simulink model "sampleModel106"  (R2022a)
settings: Solver=VariableStepAuto  StartTime=0.0  StopTime=10.0  RelTol=1e-3
undefined symbols (not defined in the file): DiscIntNeverNeededParam, magnitude, Newton, Raphson
libraries: simulink x379, slpidlib x89
(part 1 of 16)
settings Model: Creator=user  LastModifiedBy=CMelt
settings SolverCC: ZeroCrossControl=DisableAll

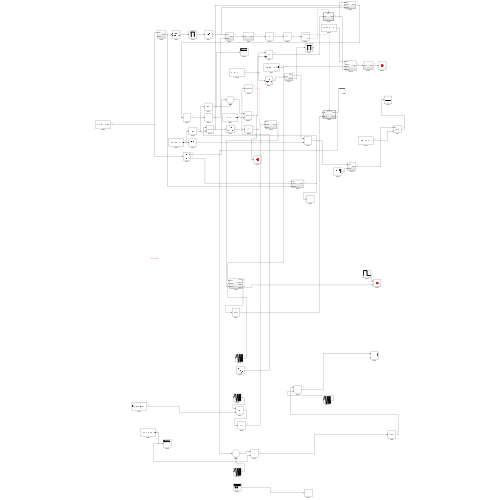
[thumbnail: Simulink's stored preview of the top-level diagram]
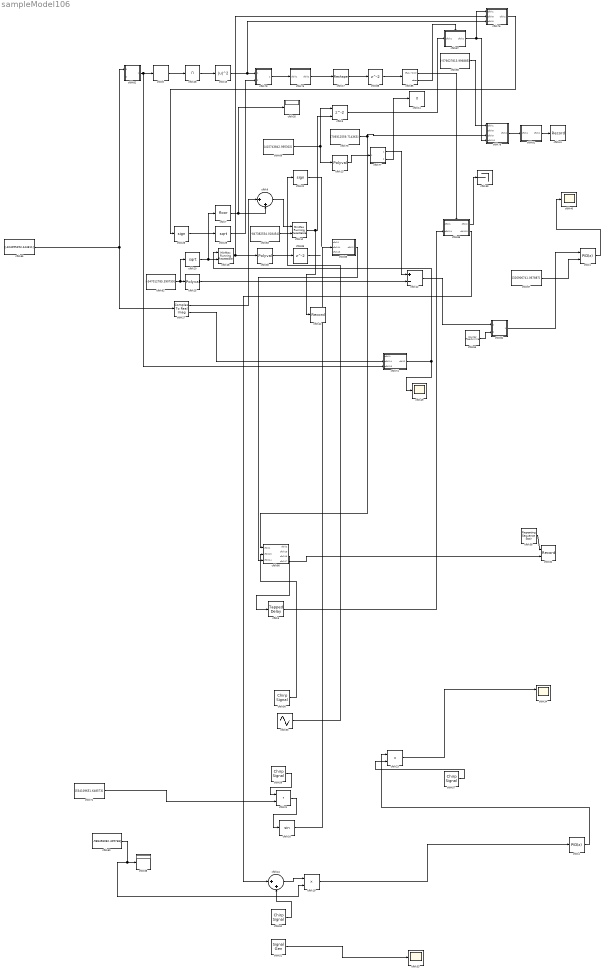
== system sampleModel106 ==
  cfblk1 : slpidlib/PID Controller (2DOF)  Controller=PID  Form=Parallel  TimeDomain=Discrete-time  UseExternalTs=off  SampleTime=1  IntegratorMethod=Forward Euler  FilterMethod=Forward Euler  ControllerParametersSource=internal  P=1  I=1  UseKiTs=off  D=0  N=100  UseFilter=on  b=1  c=1  TunerSelectOption=Transfer Function Based (PID Tuner App)  InitialConditionSource=internal  InitialConditionForIntegrator=0  InitialConditionForFilter=0  DifferentiatorICPrevScaledInput=0  ExternalReset=none  TrackingMode=off  Kt=1  LimitOutput=off  SatLimitsSource=internal  UpperSaturationLimit=inf  LowerSaturationLimit=-inf  LinearizeAsGain=off  AntiWindupMode=none  Kb=1  POutMin=[]  POutMax=[]  IOutMin=[]  IOutMax=[]  DOutMin=[]  DOutMax=[]  NOutMin=[]  NOutMax=[]  bOutMin=[]  bOutMax=[]  cOutMin=[]  cOutMax=[]  SumOutMin=[]  SumOutMax=[]  SaturationOutMin=[]  SaturationOutMax=[]  PParamMin=[]  PParamMax=[]  IParamMin=[]  IParamMax=[]  DParamMin=[]  DParamMax=[]  NParamMin=[]  NParamMax=[]  bParamMin=[]  bParamMax=[]  cParamMin=[]  cParamMax=[]  KbParamMin=[]  KbParamMax=[]  KtParamMin=[]  KtParamMax=[]  KbOutMin=[]  KbOutMax=[]  KtOutMin=[]  KtOutMax=[]  IntegratorOutMin=[]  IntegratorOutMax=[]  FilterOutMin=[]  FilterOutMax=[]  SumI1OutMin=[]  SumI1OutMax=[]  SumI2OutMin=[]  SumI2OutMax=[]  SumI3OutMin=[]  SumI3OutMax=[]  SumI4OutMin=[]  SumI4OutMax=[]  SumDOutMin=[]  SumDOutMax=[]  Sum1OutMin=[]  Sum1OutMax=[]  Sum2OutMin=[]  Sum2OutMax=[]  Sum3OutMin=[]  Sum3OutMax=[]  DifferentiatorOutMin=[]  DifferentiatorOutMax=[]  FilterDiffOutCoefMin=[]  FilterDiffOutCoefMax=[]  ReciprocalOutMin=[]  ReciprocalOutMax=[]  SumDenOutMin=[]  SumDenOutMax=[]  SumNumOutMin=[]  SumNumOutMax=[]  DivideOutMin=[]  DivideOutMax=[]  UdiffTsProdOutMin=[]  UdiffTsProdOutMax=[]  NTsProdOutMin=[]  NTsProdOutMax=[]  UintegralTsProdOutMin=[]  UintegralTsProdOutMax=[]  UngainTsProdOutMin=[]  UngainTsProdOutMax=[]  IntegratorContinuousStateAttributes=''  IntegratorStateMustResolveToSignalObject=off  IntegratorRTWStateStorageClass=Auto  FilterContinuousStateAttributes=''  FilterStateMustResolveToSignalObject=off  FilterRTWStateStorageClass=Auto  ParallelPVariant=InternalParameters  IdealPVariant=Disabled  IVariant=InternalParameters  DVariant=InternalParameters  bVariant=InternalParameters  cVariant=InternalParameters  IntegratorVariant=Discrete  SatVariant=Disabled  AWVariant=Passthrough  PCopyVariant=Disabled  TRVariant=Disabled  FdbkBlocksVariant=Forward  IdealPFdbkVariant=Disabled  SatFdbkVariant=Disabled  DerivativeFilterVariant=ForwardEulerFilter  NVariant=InternalParameters  NCopyVariant=Disabled  FilterICVariant=InternalICsFilter  IntegratorICVariant=InternalICs  ExternalResetVariant=Disabled  TRSumVariant=Passthrough  SumFdbkVariant=Disabled  SumVariant=Sum_PID  TsampFilterVariant=InternalTs  TsampNgainVariant=Passthrough  TsampIntegralVariant=Passthrough  ExternalSaturationOutDataTypeStr=Inherit: Same as second input
      settings: SourceProductBaseCode=SL
  cfblk10 : simulink/Math Operations/MinMax Running Resettable  Function=min  vinit=0.0
  cfblk11 : Product  Inputs=*
  cfblk12 : Sum  Inputs=+-
  cfblk13 : Polyval  Coefs=[ +2.081618890e-019, -1.441693666e-014, +4.719686976e-010, -8.536869453e-006, +1.621573104e-001, -8.087801117e+001 ]
  cfblk15 : Math  Operator=magnitude^2
  cfblk16 : Trigonometry
  cfblk17 : Reshape
  cfblk18 : simulink/Math Operations/MinMax Running Resettable  Function=min  vinit=0.0
  cfblk19 : Product  Inputs=**
  cfblk20 : Sqrt
  cfblk21 : DotProduct  OutDataTypeStr=Inherit: Inherit via internal rule
  cfblk22 : Signum
  cfblk23 : Product  Inputs=**
  cfblk24 : Sum  Inputs=|++
  cfblk25 : Polyval  Coefs=[ +2.081618890e-019, -1.441693666e-014, +4.719686976e-010, -8.536869453e-006, +1.621573104e-001, -8.087801117e+001 ]
  cfblk26 : Signum
  cfblk27 : ComplexToRealImag
  cfblk28 : Product  Inputs=*
  cfblk29 : Sqrt
  cfblk3 : Delay  ShowEnablePort=on  SampleTime=1
      settings: InputPortMap=u0,e6
  cfblk30 : Polyval  Coefs=[ +2.081618890e-019, -1.441693666e-014, +4.719686976e-010, -8.536869453e-006, +1.621573104e-001, -8.087801117e+001 ]
  cfblk32 : Record  FileSettingsInternal="{\"entries\":[{\"content\":{\"excelSettings\":{\"content\":{},\"type\":\"Streamout.ExcelSettings\"}},\"type\":\"Streamout.FileSettingStorage\",\"uuid\":\"e110163f-17d1-468f-aa8a-8df89c780f5b\"}],\"packageUris\":[\"http://schema.mathworks.com/mf0/streamout_blocks/R2020a\"],\"version\":\"1.0\"}"  Layout=[1 1]  SignalsInternal="{\"entries\":[{\"content\":{\"signals\":[{\"content\":{\"blockPath\":[\"sampleModel106/cfblk32\"],\"channel\":[],\"dimensions\":[1],\"domain\":\"sampleModel106/cfblk32\",\"lineColor\":\"#a2142f\",\"plots\":[],\"port\":1,\"sid\":[\"\"],\"signalID\":80912,\"signalName\":\"cfblk58\"},\"type\":\"RecordBlkView.Signal\",\"uuid\":\"457845e8-4f3e-44d6-8731-a8e61b6cf7c8\"},{\"content\":{\"blockPath\":[\"sampleModel106/cfblk32\"],\"channel\":[],\"dimensions\":[1],\"domain\":\"sampleModel106/cfblk32\",\"lineColor\":\"#139fff\",\"plots\":[],\"port\":2,\"sid\":[\"\"],\"signalID\":80916,\"signalName\":\"cfblk80:4\"},\"type\":\"RecordBlkView.Signal\",\"uuid\":\"b96e6444-998c-44db-b2f2-f137ae476481\"}]},\"type\":\"RecordBlkView.InputSignals\",\"uuid\":\"14237e14-704e-401d-9722-b40b1232ab5b\"}],\"packageUris\":[\"http://schema.mathworks.com/mf0/streamout_blocks/R2020a\"],\"version\":\"1.0\"}"  VisualizationBindings="{\"xyplotplugin\":{\"info\":[{\"series\":[],\"subplotID\":1}]}}"  CompatibilityTag=XY
  cfblk33 : Scope
  cfblk34 : Scope  NumInputPorts=2
  cfblk35 : Display
  cfblk38 : Display
  cfblk39 : Terminator
  cfblk4 : slpidlib/PID Controller  Controller=PID  Form=Parallel  TimeDomain=Discrete-time  UseExternalTs=off  SampleTime=1  IntegratorMethod=Forward Euler  FilterMethod=Forward Euler  ControllerParametersSource=internal  P=1  I=1  UseKiTs=off  D=0  N=100  UseFilter=on  TunerSelectOption=Transfer Function Based (PID Tuner App)  InitialConditionSource=internal  InitialConditionForIntegrator=0  InitialConditionForFilter=0  DifferentiatorICPrevScaledInput=0  ExternalReset=none  TrackingMode=off  Kt=1  LimitOutput=off  SatLimitsSource=internal  UpperSaturationLimit=inf  LowerSaturationLimit=-inf  LinearizeAsGain=off  AntiWindupMode=none  Kb=1  POutMin=[]  POutMax=[]  IOutMin=[]  IOutMax=[]  DOutMin=[]  DOutMax=[]  NOutMin=[]  NOutMax=[]  SumOutMin=[]  SumOutMax=[]  SaturationOutMin=[]  SaturationOutMax=[]  PParamMin=[]  PParamMax=[]  IParamMin=[]  IParamMax=[]  DParamMin=[]  DParamMax=[]  NParamMin=[]  NParamMax=[]  KbParamMin=[]  KbParamMax=[]  KtParamMin=[]  KtParamMax=[]  KbOutMin=[]  KbOutMax=[]  KtOutMin=[]  KtOutMax=[]  IntegratorOutMin=[]  IntegratorOutMax=[]  FilterOutMin=[]  FilterOutMax=[]  SumI1OutMin=[]  SumI1OutMax=[]  SumI2OutMin=[]  SumI2OutMax=[]  SumI3OutMin=[]  SumI3OutMax=[]  SumI4OutMin=[]  SumI4OutMax=[]  SumDOutMin=[]  SumDOutMax=[]  DifferentiatorOutMin=[]  DifferentiatorOutMax=[]  FilterDiffOutCoefMin=[]  FilterDiffOutCoefMax=[]  ReciprocalOutMin=[]  ReciprocalOutMax=[]  SumDenOutMin=[]  SumDenOutMax=[]  SumNumOutMin=[]  SumNumOutMax=[]  DivideOutMin=[]  DivideOutMax=[]  UdiffTsProdOutMin=[]  UdiffTsProdOutMax=[]  NTsProdOutMin=[]  NTsProdOutMax=[]  UintegralTsProdOutMin=[]  UintegralTsProdOutMax=[]  UngainTsProdOutMin=[]  UngainTsProdOutMax=[]  IntegratorContinuousStateAttributes=''  IntegratorStateMustResolveToSignalObject=off  IntegratorRTWStateStorageClass=Auto  FilterContinuousStateAttributes=''  FilterStateMustResolveToSignalObject=off  FilterRTWStateStorageClass=Auto  ParallelPVariant=InternalParameters  IdealPVariant=Disabled  IVariant=InternalParameters  DVariant=InternalParameters  IntegratorVariant=Discrete  SatVariant=Disabled  AWVariant=Passthrough  PCopyVariant=Disabled  TRVariant=Disabled  FdbkBlocksVariant=Forward  IdealPFdbkVariant=Disabled  SatFdbkVariant=Disabled  DerivativeFilterVariant=ForwardEulerFilter  NVariant=InternalParameters  NCopyVariant=Disabled  FilterICVariant=InternalICsFilter  IntegratorICVariant=InternalICs  ExternalResetVariant=Disabled  TRSumVariant=Passthrough  SumFdbkVariant=Disabled  SumVariant=Sum_PID  TsampFilterVariant=InternalTs  TsampNgainVariant=Passthrough  TsampIntegralVariant=Passthrough  ExternalSaturationOutDataTypeStr=Inherit: Same as second input  aMode=0
  cfblk40 : Scope
  cfblk41 : Record  FileSettingsInternal="{\"entries\":[{\"content\":{\"excelSettings\":{\"content\":{},\"type\":\"Streamout.ExcelSettings\"}},\"type\":\"Streamout.FileSettingStorage\",\"uuid\":\"cb7a01d5-6bb3-4fa1-ab59-b908f5278578\"}],\"packageUris\":[\"http://schema.mathworks.com/mf0/streamout_blocks/R2020a\"],\"version\":\"1.0\"}"  Layout=[1 1]  SignalsInternal="{\"entries\":[{\"content\":{\"signals\":[{\"content\":{\"blockPath\":[\"sampleModel106/cfblk41\"],\"channel\":[],\"dimensions\":[1],\"domain\":\"sampleModel106/cfblk41\",\"lineColor\":\"#77ac30\",\"plots\":[],\"port\":1,\"sid\":[\"\"],\"signalID\":80904,\"signalName\":\"cfblk81\"},\"type\":\"RecordBlkView.Signal\",\"uuid\":\"1b597b26-609b-45e7-870d-f5a73ce23ff1\"}]},\"type\":\"RecordBlkView.InputSignals\",\"uuid\":\"6f1bdcf3-e232-4e2f-ae14-9a8cce83fc18\"}],\"packageUris\":[\"http://schema.mathworks.com/mf0/streamout_blocks/R2020a\"],\"version\":\"1.0\"}"  VisualizationBindings="{\"sparklinesplugin\":{\"info\":[{\"bindingParametersList\":[],\"subplotID\":1}]}}"
  cfblk42 : Record  FileSettingsInternal="{\"entries\":[{\"content\":{\"excelSettings\":{\"content\":{},\"type\":\"Streamout.ExcelSettings\"}},\"type\":\"Streamout.FileSettingStorage\",\"uuid\":\"a4909d67-4480-489f-b4b0-8de0d839718a\"}],\"packageUris\":[\"http://schema.mathworks.com/mf0/streamout_blocks/R2020a\"],\"version\":\"1.0\"}"  Layout=[1 1]  SignalsInternal="{\"entries\":[{\"content\":{\"signals\":[{\"content\":{\"blockPath\":[\"sampleModel106/cfblk42\"],\"channel\":[],\"dimensions\":[1],\"domain\":\"sampleModel106/cfblk42\",\"lineColor\":\"#4dbeee\",\"plots\":[],\"port\":1,\"sid\":[\"\"],\"signalID\":80908,\"signalName\":\"cfblk10\"},\"type\":\"RecordBlkView.Signal\",\"uuid\":\"152f530a-83a1-42ed-a122-aabd1f7e579c\"}]},\"type\":\"RecordBlkView.InputSignals\",\"uuid\":\"05e10149-8bbc-4e26-aac1-875f3d1f5966\"}],\"packageUris\":[\"http://schema.mathworks.com/mf0/streamout_blocks/R2020a\"],\"version\":\"1.0\"}"  VisualizationBindings="{\"sparklinesplugin\":{\"info\":[{\"bindingParametersList\":[],\"subplotID\":1}]}}"
  cfblk49 : Scope
  cfblk5 : simulink/Discrete/Tapped Delay  vinit=0.0  samptime=-1  NumDelays=1  DelayOrder=Oldest  includeCurrent=off
  cfblk51 : SignalGenerator  WaveForm=sawtooth  Amplitude=[-212533553.298796]  Units=rad/sec
  cfblk52 : simulink/Sources/Chirp Signal  f1=[613766940.785120]  T=[-395095631.860066]  f2=[-802426930.856558]
  cfblk53 : Sin  Amplitude=[288589393.086639]  Bias=[-913459720.963604]  SampleTime=0
  cfblk55 : simulink/Sources/Counter Free-Running  NumBits=[55.000000]  tsamp=-1
  cfblk56 : simulink/Sources/Chirp Signal  f1=[-54418172.777980]  T=[449973931.943895]  f2=[-505913223.671693]
  cfblk57 : simulink/Sources/Chirp Signal  f1=[-525143795.572167]  T=[-268287948.430426]  f2=[-119164762.351629]
  cfblk58 : simulink/Sources/Repeating Sequence Stair  OutValues=[-775503684.180385, -893100635.461629]  tsamp=-1  OutMin=[]  OutMax=[]  OutDataTypeStr=double  OutputDataTypeScalingMode=double  OutDataType=fixdt(0,8)  ConRadixGroup=Best Precision: Vector-wise  OutScaling=2^-12
  cfblk59 : simulink/Sources/Chirp Signal  f1=[594505458.550194]  T=[-353462079.980652]  f2=[-33153660.477824]
  cfblk6 : DiscreteStateSpace
  cfblk60 : Constant  Value=[-988458082.409768]  SampleTime=1
  cfblk62 : Constant  Value=[-347012785.390759]  SampleTime=1
  cfblk63 : Constant  Value=[-847382534.018454]  SampleTime=1
  cfblk65 : Constant  Value=[-404095493.444811]  SampleTime=1
  cfblk66 : Constant  Value=[-576627813.996885]  SampleTime=1
  cfblk67 : Constant  Value=[326906741.067887]  SampleTime=1
  cfblk69 : Constant  Value=[415743842.995302]  SampleTime=1
  cfblk7 : Rounding
  cfblk71 : Constant  Value=[534109651.648573]  SampleTime=1
  cfblk73 : Constant  Value=[709312559.714363]  SampleTime=1
  cfblk74 : Subsystem
  cfblk75 : Subsystem
  cfblk76 : Subsystem
  cfblk77 : Subsystem
  cfblk78 : Subsystem
  cfblk79 : Subsystem
  cfblk80 : Subsystem
  cfblk81 : Subsystem
  cfblk82 : Subsystem
  cfblk83 : Subsystem
  cfblk84 : Subsystem
  cfblk85 : If  IfExpression=u1 >= 0  SampleTime=1
  cfblk86 : Subsystem  TreatAsAtomicUnit=on
  cfblk87 : Subsystem  TreatAsAtomicUnit=on
  cfblk88 : Delay  SampleTime=1
  cfblk89 : Delay  SampleTime=1
  cfblk9 : Sum  Inputs=|++
  wires:
  cfblk89/1 -> ?
  cfblk30/1 -> cfblk89/1
  cfblk88/1 -> cfblk85/1
  cfblk76/1(cfblk2) -> cfblk26/1
  cfblk17/1 -> cfblk88/1
  cfblk5/1 -> cfblk86/2(cfblk14)
  cfblk85/2 -> cfblk87/Action
  cfblk85/1 -> cfblk86/Action
  cfblk58/1 -> cfblk32/1
  cfblk59/1 -> cfblk21/1
  cfblk80/4(cfblk17) -> cfblk32/2
  cfblk71/1 -> cfblk21/2
  cfblk83/1(cfblk2) -> cfblk80/3(cfblk14)
  cfblk63/1 -> cfblk10/2
  cfblk27/1 -> cfblk9/1
  cfblk80/3(cfblk16) -> cfblk5/1
  cfblk52/1 -> cfblk24/2
  cfblk86/1(cfblk2) -> cfblk39/1
  cfblk27/2 -> cfblk74/2(cfblk14)
  cfblk77/2(cfblk10) -> cfblk11/1
  cfblk75/1(cfblk2) -> cfblk17/1
  cfblk9/1 -> cfblk10/1
  cfblk29/1 -> cfblk79/2(cfblk9)
  cfblk26/1 -> cfblk29/1
  cfblk57/1 -> cfblk23/2
  cfblk79/1(cfblk2) -> cfblk75/1(cfblk1)
  cfblk56/1 -> cfblk80/2(cfblk13)
  cfblk86/2(cfblk15) -> cfblk24/1
  cfblk3/1 -> cfblk87/1(cfblk1)
  cfblk65/1 -> cfblk27/1, cfblk82/1(cfblk1)
  cfblk13/1 -> cfblk77/1(cfblk1)
  cfblk4/1 -> cfblk23/1
  cfblk15/1 -> cfblk79/1(cfblk1), cfblk76/3(cfblk9)
  cfblk1/1 -> cfblk40/1
  cfblk25/1 -> cfblk12/2
  ? -> ?
  cfblk55/1 -> cfblk84/2(cfblk8)
  cfblk12/1 -> cfblk84/1(cfblk1)
  cfblk51/1 -> cfblk33/1
  cfblk66/1 -> cfblk78/1(cfblk1)
  cfblk67/1 -> cfblk1/2
  cfblk24/1 -> cfblk19/1
  cfblk23/1 -> cfblk34/1
  cfblk28/1 -> cfblk15/1
  cfblk77/1(cfblk2) -> cfblk12/1
  cfblk53/1 -> cfblk22/1
  cfblk84/1(cfblk2) -> cfblk1/1
  cfblk21/1 -> cfblk16/1
  cfblk22/1 -> ?
  cfblk78/1(cfblk2) -> cfblk81/1(cfblk1)
  cfblk19/1 -> cfblk4/1
  cfblk6/1 -> cfblk28/1
  cfblk81/1(cfblk2) -> cfblk41/1
  cfblk18/1 -> cfblk30/1, cfblk76/2(cfblk8)
  cfblk87/1(cfblk2) -> cfblk76/1(cfblk1), cfblk78/4(cfblk10)
  cfblk7/1 -> cfblk35/1, cfblk9/2
  cfblk69/1 -> cfblk13/1, cfblk3/1
  cfblk82/1(cfblk2) -> cfblk6/1, cfblk74/3(cfblk15)
  cfblk62/1 -> cfblk25/1, cfblk20/1
  cfblk16/1 -> cfblk83/2(cfblk14)
  cfblk20/1 -> cfblk18/2, cfblk7/1
  cfblk74/1(cfblk2) -> cfblk49/1, cfblk18/1
  cfblk10/1 -> cfblk42/1, cfblk3/2
  cfblk60/1 -> cfblk19/2, cfblk38/1
  cfblk73/1 -> cfblk80/1(cfblk1), cfblk78/3(cfblk9)

== system sampleModel106/cfblk74 ==
  cfblk1 : Inport
  cfblk14 : Inport  Port=2
  cfblk15 : Inport  Port=3
  cfblk10 : Subsystem
  cfblk11 : Subsystem
  cfblk12 : Subsystem
  cfblk13 : Subsystem
  cfblk16 : Delay  SampleTime=1
  cfblk17 : Delay  SampleTime=1
  cfblk18 : Delay  SampleTime=1
  cfblk3 : Sum  Inputs=+-
  cfblk4 : Sum  Inputs=+-
  cfblk5 : Assignment  DiagnosticForDimensions=Warning  IndexOptions=Index vector (dialog)  Indices=1  OutputSizes=1
  cfblk6 : Sum  Inputs=+-
  cfblk7 : MinMax  Function=max
  cfblk8 : Constant  Value=[364868605.972115]  SampleTime=1
  cfblk9 : Subsystem
  cfblk2 : Outport
  wires:
  cfblk9/1(cfblk2) -> cfblk12/1(cfblk1), cfblk11/2(cfblk7)
  cfblk5/1 -> cfblk6/1
  cfblk3/1 -> cfblk10/1(cfblk1), cfblk11/1(cfblk1)
  cfblk4/1 -> cfblk5/1
  cfblk1/1 -> cfblk9/1(cfblk1), cfblk11/3(cfblk8)
  cfblk7/1 -> cfblk3/1, cfblk4/2
  cfblk14/1 -> cfblk9/2(cfblk17)
  cfblk15/1 -> cfblk12/2(cfblk9)
  cfblk11/1(cfblk2) -> cfblk13/1(cfblk1)
  cfblk13/2(cfblk16) -> cfblk5/2
  cfblk11/2(cfblk9) -> cfblk2/1
  cfblk12/1(cfblk2) -> cfblk7/1
  cfblk12/2(cfblk10) -> cfblk13/2(cfblk14)
  cfblk8/1 -> cfblk6/2
  cfblk10/1(cfblk2) -> cfblk13/3(cfblk15)
  cfblk10/2(cfblk14) -> cfblk4/1
  cfblk13/1(cfblk2) -> cfblk16/1
  cfblk16/1 -> cfblk10/3(cfblk13)
  cfblk6/1 -> cfblk17/1
  cfblk17/1 -> cfblk10/2(cfblk12)
  cfblk13/3(cfblk17) -> cfblk18/1
  cfblk18/1 -> cfblk3/2

== system sampleModel106/cfblk75 ==
  cfblk1 : Inport
  cfblk10 : Delay  SampleTime=1
  cfblk3 : Delay  DelayLengthSource=Input port  SampleTime=1
      settings: InputPortMap=u0,p1
  cfblk4 : MinMax
  cfblk5 : Subsystem
  cfblk6 : Subsystem
  cfblk7 : Subsystem
  cfblk8 : Delay  SampleTime=1
  cfblk9 : Delay  SampleTime=1
  cfblk2 : Outport
  wires:
  cfblk4/1 -> cfblk3/1
  cfblk5/1(cfblk2) -> cfblk2/1
  cfblk7/1(cfblk2) -> cfblk4/1
  cfblk5/2(cfblk13) -> cfblk7/1(cfblk1)
  cfblk1/1 -> cfblk6/2(cfblk9), cfblk3/2
  cfblk6/1(cfblk2) -> cfblk5/1(cfblk1)
  cfblk6/2(cfblk11) -> cfblk7/2(cfblk11)
  cfblk3/1 -> cfblk8/1
  cfblk8/1 -> cfblk6/1(cfblk1)
  cfblk7/2(cfblk12) -> cfblk9/1
  cfblk9/1 -> cfblk5/2(cfblk12)
  cfblk5/3(cfblk14) -> cfblk10/1
  cfblk10/1 -> cfblk6/3(cfblk10)

== system sampleModel106/cfblk76 ==
  cfblk1 : Inport
  cfblk8 : Inport  Port=2
  cfblk9 : Inport  Port=3
  cfblk10 : Delay  SampleTime=1
  cfblk3 : Sum  Inputs=+
  cfblk4 : Subsystem
  cfblk5 : Subsystem
  cfblk6 : Subsystem
  cfblk7 : Subsystem
  cfblk2 : Outport
  wires:
  cfblk1/1 -> cfblk4/1(cfblk1), cfblk7/5(cfblk12)
  cfblk3/1 -> cfblk2/1
  cfblk7/1(cfblk2) -> cfblk5/1(cfblk1)
  cfblk6/1(cfblk2) -> cfblk7/1(cfblk1), cfblk7/3(cfblk10), cfblk7/4(cfblk11)
  cfblk4/1(cfblk2) -> cfblk5/2(cfblk7)
  cfblk8/1 -> cfblk7/2(cfblk9), cfblk6/1(cfblk1)
  cfblk9/1 -> cfblk3/1
  cfblk5/1(cfblk2) -> cfblk10/1
  cfblk10/1 -> cfblk4/2(cfblk11)

== system sampleModel106/cfblk77 ==
  cfblk1 : Inport
  cfblk11 : Subsystem  TreatAsAtomicUnit=on
  cfblk12 : Subsystem  TreatAsAtomicUnit=on
  cfblk3 : UnitDelay  HasFrameUpgradeWarning=on
  cfblk4 : simulink/Math Operations/Slider Gain  gain=1  low=0  high=2
  cfblk5 : ComplexToMagnitudeAngle
  cfblk6 : MinMax  Function=max
  cfblk7 : Constant  Value=[-2848569.974406]  SampleTime=1
  cfblk8 : Constant  Value=[-991286230.767079]  SampleTime=1
  cfblk9 : If  IfExpression=u1 >= 0  SampleTime=1
  cfblk2 : Outport
  cfblk10 : Outport  Port=2
  wires:
  cfblk11/1(cfblk2) -> cfblk4/1
  cfblk3/1 -> cfblk10/1
  cfblk4/1 -> cfblk6/1
  cfblk7/1 -> cfblk9/1
  cfblk8/1 -> cfblk11/1(cfblk1)
  cfblk5/1 -> cfblk12/1(cfblk1)
  cfblk5/2 -> cfblk2/1
  cfblk12/1(cfblk2) -> cfblk11/2(cfblk7)
  cfblk12/2(cfblk7) -> cfblk11/3(cfblk8), cfblk11/5(cfblk10)
  cfblk1/1 -> cfblk5/1, cfblk11/4(cfblk9)
  cfblk6/1 -> cfblk3/1
  cfblk9/1 -> cfblk11/Action
  cfblk9/2 -> cfblk12/Action

== system sampleModel106/cfblk78 ==
  cfblk1 : Inport
  cfblk8 : Inport  Port=2
  cfblk9 : Inport  Port=3
  cfblk10 : Inport  Port=4
  cfblk11 : Subsystem  TreatAsAtomicUnit=on
  cfblk12 : Subsystem  TreatAsAtomicUnit=on
  cfblk3 : simulink/Discrete/Transfer Fcn Lead or Lag  PoleZ=0.95  ZeroZ=0.75  ICPrevOutput=0.0  ICPrevInput=0.0  DoSatur=off
      settings: SourceProductBaseCode=SL
  cfblk4 : Bias  Bias=[142934290.678722]  SaturateOnIntegerOverflow=off
  cfblk5 : Constant  Value=[727121668.085186]  SampleTime=1
  cfblk6 : Constant  Value=[335181993.048413]  SampleTime=1
  cfblk7 : If  IfExpression=u1 >= 0  SampleTime=1
  cfblk2 : Outport
  wires:
  cfblk9/1 -> cfblk11/1(cfblk1)
  cfblk3/1 -> cfblk12/1(cfblk1)
  cfblk4/1 -> cfblk2/1
  cfblk6/1 -> cfblk3/1
  cfblk8/1 -> cfblk12/2(cfblk6)
  cfblk5/1 -> cfblk7/1
  cfblk1/1 -> cfblk4/1
  cfblk10/1 -> cfblk11/2(cfblk8)
  cfblk12/1(cfblk2) -> cfblk11/3(cfblk9)
  cfblk7/1 -> cfblk11/Action
  cfblk7/2 -> cfblk12/Action

== system sampleModel106/cfblk79 ==
  cfblk1 : Inport
  cfblk9 : Inport  Port=2
  cfblk10 : Delay  SampleTime=1
  cfblk3 : simulink/Discrete/Tapped Delay  vinit=0.0  samptime=-1  NumDelays=1  DelayOrder=Oldest  includeCurrent=off
  cfblk4 : MinMax  Function=max  Inputs=2
  cfblk5 : Bias  Bias=[-456455561.648112]  SaturateOnIntegerOverflow=off
  cfblk6 : Subsystem
  cfblk7 : Subsystem
  cfblk8 : Subsystem
  cfblk2 : Outport
  wires:
  cfblk8/1(cfblk2) -> cfblk7/1(cfblk1), cfblk10/1
  cfblk9/1 -> cfblk6/1(cfblk1)
  cfblk7/1(cfblk2) -> cfblk2/1
  cfblk6/1(cfblk2) -> cfblk7/2(cfblk14)
  cfblk5/1 -> cfblk4/1
  cfblk3/1 -> cfblk5/1
  cfblk1/1 -> cfblk3/1, cfblk7/3(cfblk15)
  cfblk4/1 -> cfblk8/1(cfblk1)
  cfblk10/1 -> cfblk4/2

== system sampleModel106/cfblk80 ==
  cfblk1 : Inport
  cfblk13 : Inport  Port=2
  cfblk14 : Inport  Port=3
  cfblk10 : Subsystem
  cfblk11 : Subsystem
  cfblk12 : Subsystem
  cfblk{18..21} (4 alike) : Delay  SampleTime=1
  cfblk3 : DiscreteTransferFcn  SampleTime=1
  cfblk4 : PermuteDimensions
  cfblk5 : MinMax
  cfblk6 : Assignment  DiagnosticForDimensions=Warning  IndexOptions=Index vector (dialog)  Indices=1  OutputSizes=1
  cfblk7 : Constant  Value=[-128863520.704600]  SampleTime=1
  cfblk8 : Subsystem
  cfblk9 : Subsystem
  cfblk2 : Outport
  cfblk15 : Outport  Port=2
  cfblk16 : Outport  Port=3
  cfblk17 : Outport  Port=4
  wires:
  cfblk13/1 -> cfblk16/1
  cfblk1/1 -> cfblk15/1, cfblk11/3(cfblk12)
  cfblk5/1 -> cfblk8/3(cfblk10), cfblk8/4(cfblk11), cfblk18/1
  cfblk10/1(cfblk2) -> cfblk3/1
  cfblk4/1 -> cfblk10/1(cfblk1), cfblk12/3(cfblk11)
  cfblk8/1(cfblk2) -> cfblk19/1, cfblk20/1
  cfblk7/1 -> cfblk4/1, cfblk9/2(cfblk8)
  cfblk6/1 -> cfblk12/1(cfblk1)
  cfblk12/1(cfblk2) -> cfblk5/1
  cfblk9/1(cfblk2) -> cfblk6/2
  cfblk11/1(cfblk2) -> cfblk17/1
  cfblk14/1 -> cfblk8/1(cfblk1)
  cfblk11/2(cfblk13) -> cfblk9/1(cfblk1)
  cfblk12/2(cfblk12) -> cfblk8/2(cfblk9)
  cfblk9/2(cfblk9) -> cfblk10/3(cfblk15)
  cfblk11/3(cfblk14) -> cfblk2/1
  cfblk9/3(cfblk10) -> cfblk12/2(cfblk10)
  cfblk18/1 -> cfblk6/1
  cfblk19/1 -> cfblk11/1(cfblk1)
  cfblk20/1 -> cfblk11/2(cfblk11)
  cfblk3/1 -> cfblk21/1
  cfblk21/1 -> cfblk10/2(cfblk14)

== system sampleModel106/cfblk81 ==
  cfblk1 : Inport
  cfblk3 : DiscreteFilter  SampleTime=1
  cfblk4 : Abs  SaturateOnIntegerOverflow=off
  cfblk5 : Constant  Value=[-416387386.623722]  SampleTime=1
  cfblk6 : Constant  Value=[865158828.827194]  SampleTime=1
  cfblk7 : Constant  Value=[47616444.552319]  SampleTime=1
  cfblk8 : Subsystem
  cfblk2 : Outport
  wires:
  cfblk5/1 -> cfblk4/1
  cfblk4/1 -> cfblk2/1
  cfblk7/1 -> cfblk8/1(cfblk1), cfblk8/4(cfblk9)
  cfblk1/1 -> cfblk3/1, cfblk8/5(cfblk10)
  cfblk6/1 -> cfblk8/2(cfblk7)
  cfblk3/1 -> cfblk8/3(cfblk8)

== system sampleModel106/cfblk82 ==
  cfblk1 : Inport
  cfblk9 : Inport  Port=2
  cfblk10 : Delay  SampleTime=1
  cfblk11 : Delay  SampleTime=1
  cfblk3 : simulink/Discrete/Tapped Delay  vinit=0.0  samptime=-1  NumDelays=1  DelayOrder=Oldest  includeCurrent=off
  cfblk4 : Polyval  Coefs=[ +2.081618890e-019, -1.441693666e-014, +4.719686976e-010, -8.536869453e-006, +1.621573104e-001, -8.087801117e+001 ]
  cfblk5 : MinMax  Function=max  Inputs=3
  cfblk6 : Sum  Inputs=+
  cfblk7 : Subsystem
  cfblk8 : Subsystem
  cfblk2 : Outport
  wires:
  cfblk1/1 -> cfblk8/1(cfblk1), cfblk6/1, cfblk7/3(cfblk11)
  cfblk5/1 -> cfblk4/1
  cfblk9/1 -> cfblk7/1(cfblk1)
  cfblk8/1(cfblk2) -> cfblk5/2
  cfblk6/1 -> cfblk2/1, cfblk5/3
  cfblk4/1 -> cfblk3/1, cfblk7/2(cfblk10)
  cfblk3/1 -> cfblk10/1
  cfblk10/1 -> cfblk5/1
  cfblk7/1(cfblk2) -> cfblk11/1
  cfblk11/1 -> cfblk8/2(cfblk11)

== system sampleModel106/cfblk83 ==
  cfblk1 : Inport
  cfblk14 : Inport  Port=2
  cfblk15 : Inport  Port=3
  cfblk10 : Constant  Value=[872034346.732977]  SampleTime=1
  cfblk11 : Subsystem
  cfblk12 : Subsystem
  cfblk13 : Subsystem
  cfblk16 : Delay  SampleTime=1
  cfblk17 : Delay  SampleTime=1
  cfblk3 : Sum
  cfblk4 : Reshape
  cfblk5 : Assignment  DiagnosticForDimensions=Warning  IndexOptions=Index vector (dialog)  Indices=1  OutputSizes=1
  cfblk6 : Abs  SaturateOnIntegerOverflow=off
  cfblk7 : Constant  Value=[391850143.586155]  SampleTime=1
  cfblk8 : Constant  Value=[472978901.667493]  SampleTime=1
  cfblk9 : Constant  Value=[705339919.245068]  SampleTime=1
  cfblk2 : Outport
  wires:
  cfblk15/1 -> cfblk5/1
  cfblk11/1(cfblk2) -> cfblk5/2
  cfblk8/1 -> cfblk13/1(cfblk1)
  cfblk14/1 -> cfblk13/2(cfblk14)
  cfblk10/1 -> cfblk6/1
  cfblk13/1(cfblk2) -> cfblk12/1(cfblk1)
  cfblk1/1 -> cfblk3/1
  cfblk11/2(cfblk14) -> cfblk13/3(cfblk15)
  cfblk6/1 -> cfblk11/1(cfblk1)
  cfblk3/1 -> cfblk11/2(cfblk12)
  cfblk9/1 -> cfblk2/1
  cfblk11/3(cfblk15) -> cfblk4/1
  cfblk5/1 -> cfblk13/4(cfblk16)
  cfblk12/1(cfblk2) -> cfblk16/1
  cfblk16/1 -> cfblk3/2
  cfblk4/1 -> cfblk17/1
  cfblk17/1 -> cfblk11/3(cfblk13)

== system sampleModel106/cfblk84 ==
  cfblk1 : Inport
  cfblk8 : Inport  Port=2
  cfblk10 : Subsystem  TreatAsAtomicUnit=on
  cfblk{11..16} (6 alike) : Delay  SampleTime=1
  cfblk3 : Sqrt  Operator=rSqrt  AlgorithmType=Newton-Raphson
  cfblk4 : PermuteDimensions
  cfblk5 : Subsystem
  cfblk6 : Subsystem
  cfblk7 : If  IfExpression=u1 >= 0  SampleTime=1
  cfblk9 : Subsystem  TreatAsAtomicUnit=on
  cfblk2 : Outport
  wires:
  cfblk6/1(cfblk2) -> cfblk7/1
  cfblk3/1 -> cfblk2/1, cfblk6/5(cfblk11)
  cfblk1/1 -> cfblk3/1, cfblk6/6(cfblk12)
  cfblk10/1(cfblk2) -> cfblk4/1, cfblk16/1
  cfblk4/1 -> cfblk5/1(cfblk1)
  cfblk8/1 -> cfblk10/1(cfblk1)
  cfblk9/1(cfblk2) -> cfblk5/2(cfblk15)
  cfblk9/2(cfblk15) -> cfblk14/1, cfblk15/1
  cfblk7/1 -> cfblk9/Action
  cfblk7/2 -> cfblk10/Action
  cfblk5/1(cfblk2) -> cfblk11/1
  cfblk11/1 -> cfblk9/1(cfblk1)
  cfblk5/2(cfblk16) -> cfblk12/1
  cfblk12/1 -> cfblk6/1(cfblk1)
  cfblk5/3(cfblk17) -> cfblk13/1
  cfblk13/1 -> cfblk9/2(cfblk14)
  cfblk14/1 -> cfblk6/2(cfblk8)
  cfblk15/1 -> cfblk6/3(cfblk9)
  cfblk16/1 -> cfblk6/4(cfblk10)

== system sampleModel106/cfblk86 ==
  cfblk1 : Inport
  cfblk14 : Inport  Port=2
  Action Port : ActionPort  ActionPortLabel=if(u1 >= 0)
  cfblk10 : Subsystem
  cfblk11 : Subsystem
  cfblk12 : Subsystem
  cfblk13 : Subsystem
  cfblk16 : Delay
  cfblk17 : Delay
  cfblk3 : slpidlib/PID Controller  Controller=PID  Form=Parallel  TimeDomain=Discrete-time  UseExternalTs=off  SampleTime=-1  IntegratorMethod=Forward Euler  FilterMethod=Forward Euler  ControllerParametersSource=internal  P=1  I=1  UseKiTs=off  D=0  N=100  UseFilter=on  TunerSelectOption=Transfer Function Based (PID Tuner App)  InitialConditionSource=internal  InitialConditionForIntegrator=0  InitialConditionForFilter=0  DifferentiatorICPrevScaledInput=0  ExternalReset=none  TrackingMode=off  Kt=1  LimitOutput=off  SatLimitsSource=internal  UpperSaturationLimit=inf  LowerSaturationLimit=-inf  LinearizeAsGain=off  AntiWindupMode=none  Kb=1  POutMin=[]  POutMax=[]  IOutMin=[]  IOutMax=[]  DOutMin=[]  DOutMax=[]  NOutMin=[]  NOutMax=[]  SumOutMin=[]  SumOutMax=[]  SaturationOutMin=[]  SaturationOutMax=[]  PParamMin=[]  PParamMax=[]  IParamMin=[]  IParamMax=[]  DParamMin=[]  DParamMax=[]  NParamMin=[]  NParamMax=[]  KbParamMin=[]  KbParamMax=[]  KtParamMin=[]  KtParamMax=[]  KbOutMin=[]  KbOutMax=[]  KtOutMin=[]  KtOutMax=[]  IntegratorOutMin=[]  IntegratorOutMax=[]  FilterOutMin=[]  FilterOutMax=[]  SumI1OutMin=[]  SumI1OutMax=[]  SumI2OutMin=[]  SumI2OutMax=[]  SumI3OutMin=[]  SumI3OutMax=[]  SumI4OutMin=[]  SumI4OutMax=[]  SumDOutMin=[]  SumDOutMax=[]  DifferentiatorOutMin=[]  DifferentiatorOutMax=[]  FilterDiffOutCoefMin=[]  FilterDiffOutCoefMax=[]  ReciprocalOutMin=[]  ReciprocalOutMax=[]  SumDenOutMin=[]  SumDenOutMax=[]  SumNumOutMin=[]  SumNumOutMax=[]  DivideOutMin=[]  DivideOutMax=[]  UdiffTsProdOutMin=[]  UdiffTsProdOutMax=[]  NTsProdOutMin=[]  NTsProdOutMax=[]  UintegralTsProdOutMin=[]  UintegralTsProdOutMax=[]  UngainTsProdOutMin=[]  UngainTsProdOutMax=[]  IntegratorContinuousStateAttributes=''  IntegratorStateMustResolveToSignalObject=off  IntegratorRTWStateStorageClass=Auto  FilterContinuousStateAttributes=''  FilterStateMustResolveToSignalObject=off  FilterRTWStateStorageClass=Auto  ParallelPVariant=InternalParameters  IdealPVariant=Disabled  IVariant=InternalParameters  DVariant=InternalParameters  IntegratorVariant=Discrete  SatVariant=Disabled  AWVariant=Passthrough  PCopyVariant=Disabled  TRVariant=Disabled  FdbkBlocksVariant=Forward  IdealPFdbkVariant=Disabled  SatFdbkVariant=Disabled  DerivativeFilterVariant=ForwardEulerFilter  NVariant=InternalParameters  NCopyVariant=Disabled  FilterICVariant=InternalICsFilter  IntegratorICVariant=InternalICs  ExternalResetVariant=Disabled  TRSumVariant=Passthrough  SumFdbkVariant=Disabled  SumVariant=Sum_PID  TsampFilterVariant=InternalTs  TsampNgainVariant=Passthrough  TsampIntegralVariant=Passthrough  ExternalSaturationOutDataTypeStr=Inherit: Same as second input  aMode=0
  cfblk4 : Delay
  cfblk5 : PermuteDimensions
  cfblk6 : ComplexToRealImag
  cfblk7 : Sin  TimeSource=Use external signal  SampleTime=0
  cfblk8 : Trigonometry
  cfblk9 : Subsystem
  cfblk2 : Outport
  cfblk15 : Outport  Port=2
  wires:
  cfblk6/1 -> cfblk7/1
  cfblk11/1(cfblk2) -> cfblk3/1
  cfblk12/1(cfblk2) -> cfblk15/1
  cfblk6/2 -> cfblk8/1
  cfblk1/1 -> cfblk11/1(cfblk1)
  cfblk3/1 -> cfblk6/1, cfblk10/3(cfblk15), cfblk9/2(cfblk9)
  cfblk7/1 -> cfblk10/1(cfblk1), cfblk9/4(cfblk11)
  cfblk14/1 -> cfblk13/1(cfblk1), cfblk10/4(cfblk16)
  cfblk10/1(cfblk2) -> cfblk4/1
  cfblk13/1(cfblk2) -> cfblk2/1
  cfblk4/1 -> cfblk12/1(cfblk1)
  cfblk8/1 -> cfblk12/2(cfblk12)
  cfblk5/1 -> cfblk16/1, cfblk17/1
  cfblk9/1(cfblk2) -> cfblk10/2(cfblk14)
  cfblk9/2(cfblk12) -> cfblk5/1
  cfblk16/1 -> cfblk9/1(cfblk1)
  cfblk17/1 -> cfblk9/3(cfblk10)

== system sampleModel106/cfblk87 ==
  cfblk1 : Inport
  Action Port : ActionPort  ActionPortLabel=else
  cfblk10 : Delay
  cfblk11 : Delay
  cfblk3 : Delay
  cfblk4 : Polyval  Coefs=[ +2.081618890e-019, -1.441693666e-014, +4.719686976e-010, -8.536869453e-006, +1.621573104e-001, -8.087801117e+001 ]
  cfblk5 : simulink/Math Operations/Slider Gain  gain=1  low=0  high=2
  cfblk6 : Assignment  DiagnosticForDimensions=Warning  IndexOptions=Index vector (dialog)  Indices=1  OutputSizes=1
  cfblk7 : Subsystem
  cfblk8 : Subsystem
  cfblk9 : Subsystem
  cfblk2 : Outport
  wires:
  cfblk7/1(cfblk2) -> cfblk4/1
  cfblk9/1(cfblk2) -> cfblk7/1(cfblk1)
  cfblk4/1 -> cfblk8/1(cfblk1)
  cfblk8/1(cfblk2) -> cfblk2/1
  cfblk3/1 -> cfblk9/1(cfblk1)
  cfblk5/1 -> cfblk6/2, cfblk7/2(cfblk12)
  cfblk1/1 -> cfblk5/1
  cfblk6/1 -> cfblk3/1, cfblk7/3(cfblk13), cfblk8/2(cfblk12)
  cfblk7/2(cfblk14) -> cfblk10/1
  cfblk10/1 -> cfblk6/1
  cfblk7/3(cfblk15) -> cfblk11/1
  cfblk11/1 -> cfblk9/2(cfblk16)

== system sampleModel106/cfblk74/cfblk10 ==
  cfblk1 : Inport
  cfblk12 : Inport  Port=2
  cfblk13 : Inport  Port=3
  cfblk10 : Constant  Value=[780676190.591761]  SampleTime=1
  cfblk11 : Subsystem
  cfblk15 : Delay  SampleTime=1
  cfblk3 : ComplexToMagnitudeAngle
  cfblk4 : Product
  cfblk5 : Sum  Inputs=|++
  cfblk6 : Sum  Inputs=|++
  cfblk7 : Constant  Value=[224077902.825236]  SampleTime=1
  cfblk8 : Constant  Value=[-875317570.421617]  SampleTime=1
  cfblk9 : Constant  Value=[-10612442.492546]  SampleTime=1
  cfblk2 : Outport
  cfblk14 : Outport  Port=2
  wires:
  cfblk12/1 -> cfblk11/1(cfblk1)
  cfblk9/1 -> cfblk6/1
  cfblk3/1 -> cfblk4/1
  cfblk3/2 -> cfblk4/2
  cfblk5/1 -> cfblk2/1
  cfblk10/1 -> cfblk5/1, cfblk11/4(cfblk15)
  cfblk13/1 -> cfblk14/1
  cfblk1/1 -> cfblk6/2
  cfblk7/1 -> cfblk5/2
  cfblk6/1 -> cfblk11/2(cfblk13)
  cfblk8/1 -> cfblk11/3(cfblk14)
  cfblk4/1 -> cfblk15/1
  cfblk15/1 -> cfblk3/1

== system sampleModel106/cfblk74/cfblk11 ==
  cfblk1 : Inport
  cfblk7 : Inport  Port=2
  cfblk8 : Inport  Port=3
  cfblk10 : Delay  SampleTime=1
  cfblk3 : simulink/Discrete/Transfer Fcn Real Zero  ZeroZ=0.75  ICPrevInput=0.0  DoSatur=off
      settings: SourceProductBaseCode=SL
  cfblk4 : Sum  Inputs=+
  cfblk5 : Constant  Value=[436597899.061060]  SampleTime=1
  cfblk6 : Subsystem
  cfblk2 : Outport
  cfblk9 : Outport  Port=2
  wires:
  cfblk1/1 -> cfblk2/1
  cfblk8/1 -> cfblk4/1
  cfblk5/1 -> cfblk6/1(cfblk1)
  cfblk7/1 -> cfblk6/2(cfblk12)
  cfblk4/1 -> cfblk6/3(cfblk13), cfblk6/5(cfblk15)
  cfblk3/1 -> cfblk9/1, cfblk6/4(cfblk14)
  cfblk6/1(cfblk2) -> cfblk10/1
  cfblk10/1 -> cfblk3/1

== system sampleModel106/cfblk74/cfblk12 ==
  cfblk1 : Inport
  cfblk9 : Inport  Port=2
  cfblk11 : Delay  SampleTime=1
  cfblk12 : Delay  SampleTime=1
  cfblk3 : DiscreteStateSpace
  cfblk4 : Abs  SaturateOnIntegerOverflow=off
  cfblk5 : Constant  Value=[-885945658.824691]  SampleTime=1
  cfblk6 : Subsystem
  cfblk7 : Subsystem
  cfblk8 : Subsystem
  cfblk2 : Outport
  cfblk10 : Outport  Port=2
  wires:
  cfblk5/1 -> cfblk10/1
  cfblk1/1 -> cfblk8/1(cfblk1), cfblk6/2(cfblk15)
  cfblk9/1 -> cfblk6/1(cfblk1)
  cfblk8/1(cfblk2) -> cfblk2/1
  cfblk8/2(cfblk12) -> cfblk3/1
  cfblk3/1 -> cfblk4/1
  cfblk8/3(cfblk13) -> cfblk7/1(cfblk1)
  cfblk6/1(cfblk2) -> cfblk8/4(cfblk11)
  cfblk4/1 -> cfblk11/1
  cfblk11/1 -> cfblk8/3(cfblk10)
  cfblk7/1(cfblk2) -> cfblk12/1
  cfblk12/1 -> cfblk8/2(cfblk9)

== system sampleModel106/cfblk74/cfblk13 ==
  cfblk1 : Inport
  cfblk14 : Inport  Port=2
  cfblk15 : Inport  Port=3
  cfblk10 : Constant  Value=[583226578.583847]  SampleTime=1
  cfblk11 : Subsystem
  cfblk12 : Subsystem
  cfblk13 : Subsystem
  cfblk{18..21} (4 alike) : Delay  SampleTime=1
  cfblk3 : Product
  cfblk4 : MinMax  Inputs=3
  cfblk5 : Sum  Inputs=--
  cfblk6 : PermuteDimensions
  cfblk7 : Gain  Gain=[-250665930.883016]
  cfblk8 : Math  Operator=10^u
  cfblk9 : Constant  Value=[-921108902.899406]  SampleTime=1
  cfblk2 : Outport
  cfblk16 : Outport  Port=2
  cfblk17 : Outport  Port=3
  wires:
  cfblk14/1 -> cfblk6/1
  cfblk7/1 -> cfblk8/1
  cfblk5/1 -> cfblk11/1(cfblk1)
  cfblk3/1 -> cfblk5/1, cfblk18/1
  cfblk9/1 -> cfblk13/2(cfblk13), cfblk2/1
  cfblk13/1(cfblk2) -> cfblk12/1(cfblk1)
  cfblk10/1 -> cfblk7/1
  cfblk1/1 -> cfblk13/3(cfblk14), cfblk5/2
  cfblk8/1 -> cfblk16/1
  cfblk12/1(cfblk2) -> cfblk3/1
  cfblk6/1 -> cfblk3/2
  cfblk11/1(cfblk2) -> cfblk17/1
  cfblk4/1 -> cfblk20/1, cfblk21/1
  cfblk11/2(cfblk13) -> cfblk4/2, cfblk19/1
  cfblk12/2(cfblk14) -> cfblk4/1
  cfblk15/1 -> cfblk12/3(cfblk12), cfblk4/3
  cfblk18/1 -> cfblk13/1(cfblk1)
  cfblk19/1 -> cfblk12/2(cfblk11)
  cfblk20/1 -> cfblk11/2(cfblk12)
  cfblk21/1 -> cfblk12/4(cfblk13)

== system sampleModel106/cfblk74/cfblk9 ==
  cfblk1 : Inport
  cfblk17 : Inport  Port=2
  cfblk10 : Subsystem
  cfblk11 : Subsystem
  cfblk12 : Subsystem
  cfblk13 : Subsystem
  cfblk14 : Subsystem
  cfblk15 : Subsystem
  cfblk16 : Subsystem
  cfblk18 : Delay  SampleTime=1
  cfblk19 : Delay  SampleTime=1
  cfblk3 : DiscreteIntegrator  ICPrevOutput=DiscIntNeverNeededParam  ICPrevScaledInput=DiscIntNeverNeededParam
  cfblk4 : DiscreteStateSpace
  cfblk5 : Reshape
  cfblk6 : Polyval  Coefs=[ +2.081618890e-019, -1.441693666e-014, +4.719686976e-010, -8.536869453e-006, +1.621573104e-001, -8.087801117e+001 ]
  cfblk7 : Sum  Inputs=+-
  cfblk8 : Constant  Value=[-591222895.532697]  SampleTime=1
  cfblk9 : Subsystem
  cfblk2 : Outport
  wires:
  cfblk14/1(cfblk2) -> cfblk16/1(cfblk1)
  cfblk16/1(cfblk2) -> cfblk2/1
  cfblk5/1 -> cfblk11/1(cfblk1)
  cfblk15/1(cfblk2) -> cfblk10/1(cfblk1)
  cfblk9/1(cfblk2) -> cfblk4/1
  cfblk7/1 -> cfblk15/1(cfblk1)
  cfblk14/2(cfblk8) -> cfblk5/1
  cfblk4/1 -> cfblk11/2(cfblk10)
  cfblk1/1 -> cfblk9/1(cfblk1)
  cfblk10/1(cfblk2) -> cfblk3/1
  cfblk14/3(cfblk9) -> cfblk13/1(cfblk1)
  cfblk14/4(cfblk10) -> cfblk9/2(cfblk12)
  cfblk8/1 -> cfblk10/2(cfblk7)
  cfblk11/1(cfblk2) -> cfblk7/1
  cfblk6/1 -> cfblk7/2
  cfblk17/1 -> cfblk14/1(cfblk1)
  cfblk16/2(cfblk9) -> cfblk6/1
  cfblk12/1(cfblk2) -> cfblk14/2(cfblk7)
  cfblk3/1 -> cfblk18/1
  cfblk18/1 -> cfblk15/2(cfblk12)
  cfblk13/1(cfblk2) -> cfblk19/1
  cfblk19/1 -> cfblk12/1(cfblk1)

== system sampleModel106/cfblk75/cfblk5 ==
  cfblk1 : Inport
  cfblk12 : Inport  Port=2
  cfblk10 : Subsystem
  cfblk11 : Subsystem
  cfblk15 : Delay  SampleTime=1
  cfblk3 : Product
  cfblk4 : Bias  Bias=[149759954.233905]  SaturateOnIntegerOverflow=off
  cfblk5 : Product  Inputs=*
  cfblk6 : Polyval  Coefs=[ +2.081618890e-019, -1.441693666e-014, +4.719686976e-010, -8.536869453e-006, +1.621573104e-001, -8.087801117e+001 ]
  cfblk7 : Gain  Gain=[-329678348.195251]
  cfblk8 : Constant  Value=[-633888942.912637]  SampleTime=1
  cfblk9 : Subsystem
  cfblk2 : Outport
  cfblk13 : Outport  Port=2
  cfblk14 : Outport  Port=3
  wires:
  cfblk9/1(cfblk2) -> cfblk10/1(cfblk1)
  cfblk3/1 -> cfblk5/1
  cfblk7/1 -> cfblk6/1, cfblk13/1
  cfblk11/1(cfblk2) -> cfblk3/2, cfblk7/1
  cfblk10/1(cfblk2) -> cfblk11/1(cfblk1)
  cfblk8/1 -> cfblk2/1
  cfblk9/2(cfblk11) -> cfblk11/2(cfblk11)
  cfblk6/1 -> cfblk14/1
  cfblk12/1 -> cfblk11/3(cfblk12)
  cfblk4/1 -> cfblk11/4(cfblk13)
  cfblk1/1 -> cfblk9/1(cfblk1), cfblk4/1
  cfblk5/1 -> cfblk15/1
  cfblk15/1 -> cfblk3/1

== system sampleModel106/cfblk75/cfblk6 ==
  cfblk1 : Inport
  cfblk9 : Inport  Port=2
  cfblk10 : Inport  Port=3
  cfblk12 : Delay  SampleTime=1
  cfblk13 : Delay  SampleTime=1
  cfblk14 : Delay  SampleTime=1
  cfblk3 : Product
  cfblk4 : Constant  Value=[-68312650.529540]  SampleTime=1
  cfblk5 : Subsystem
  cfblk6 : Subsystem
  cfblk7 : Subsystem
  cfblk8 : Subsystem
  cfblk2 : Outport
  cfblk11 : Outport  Port=2
  wires:
  cfblk10/1 -> cfblk8/1(cfblk1)
  cfblk9/1 -> cfblk8/2(cfblk13)
  cfblk6/1(cfblk2) -> cfblk11/1, cfblk8/3(cfblk14)
  cfblk5/1(cfblk2) -> cfblk3/1, cfblk6/2(cfblk15)
  cfblk8/2(cfblk15) -> cfblk2/1, cfblk14/1
  cfblk4/1 -> cfblk3/2, cfblk6/1(cfblk1), cfblk5/3(cfblk9), cfblk5/4(cfblk10)
  cfblk1/1 -> cfblk7/2(cfblk10)
  cfblk7/1(cfblk2) -> cfblk5/2(cfblk8), cfblk6/4(cfblk17)
  cfblk3/1 -> cfblk12/1
  cfblk12/1 -> cfblk7/1(cfblk1)
  cfblk8/1(cfblk2) -> cfblk13/1
  cfblk13/1 -> cfblk5/1(cfblk1)
  cfblk14/1 -> cfblk6/3(cfblk16)

== system sampleModel106/cfblk75/cfblk7 ==
  cfblk1 : Inport
  cfblk11 : Inport  Port=2
  cfblk10 : If  IfExpression=u1 >= 0  SampleTime=1
  cfblk13 : Subsystem  TreatAsAtomicUnit=on
  cfblk14 : Subsystem  TreatAsAtomicUnit=on
  cfblk{15..18} (4 alike) : Delay  SampleTime=1
  cfblk3 : simulink/Discrete/Transfer Fcn First Order  PoleZ=0.95  ICPrevOutput=0.0  DoSatur=off
  cfblk4 : Sum
  cfblk5 : Assignment  DiagnosticForDimensions=Warning  IndexOptions=Index vector (dialog)  Indices=1  OutputSizes=1
  cfblk6 : ComplexToMagnitudeAngle
  cfblk7 : Constant  Value=[994656215.102476]  SampleTime=1
  cfblk8 : Subsystem
  cfblk9 : Subsystem
  cfblk2 : Outport
  cfblk12 : Outport  Port=2
  wires:
  cfblk11/1 -> cfblk14/1(cfblk1)
  cfblk1/1 -> cfblk4/1
  cfblk5/1 -> cfblk12/1, cfblk13/3(cfblk12)
  cfblk3/1 -> cfblk10/1
  cfblk7/1 -> cfblk6/1
  cfblk13/1(cfblk2) -> cfblk9/1(cfblk1)
  cfblk13/2(cfblk13) -> cfblk2/1
  cfblk4/1 -> cfblk5/1
  cfblk6/1 -> cfblk8/1(cfblk1)
  cfblk6/2 -> cfblk8/2(cfblk11)
  cfblk8/1(cfblk2) -> cfblk13/1(cfblk1)
  cfblk8/2(cfblk12) -> cfblk9/2(cfblk8)
  cfblk10/1 -> cfblk13/Action
  cfblk10/2 -> cfblk14/Action
  cfblk9/1(cfblk2) -> cfblk15/1
  cfblk15/1 -> cfblk5/2
  cfblk9/2(cfblk9) -> cfblk16/1
  cfblk16/1 -> cfblk13/2(cfblk11)
  cfblk13/3(cfblk14) -> cfblk17/1
  cfblk17/1 -> cfblk4/2
  cfblk14/1(cfblk2) -> cfblk18/1
  cfblk18/1 -> cfblk3/1

== system sampleModel106/cfblk76/cfblk4 ==
  cfblk1 : Inport
  cfblk11 : Inport  Port=2
  cfblk10 : Subsystem
  cfblk12 : Delay  SampleTime=1
  cfblk13 : Delay  SampleTime=1
  cfblk3 : simulink/Discrete/Difference  ICPrevInput=0.0  OutMin=[]  OutMax=[]  OutDataTypeStr=Inherit: Inherit via back propagation  OutDataType=fixdt(1, 16)  OutScaling=2^-10  DoSatur=off
  cfblk4 : slpidlib/PID Controller (2DOF)  Controller=PID  Form=Parallel  TimeDomain=Discrete-time  UseExternalTs=off  SampleTime=1  IntegratorMethod=Forward Euler  FilterMethod=Forward Euler  ControllerParametersSource=internal  P=1  I=1  UseKiTs=off  D=0  N=100  UseFilter=on  b=1  c=1  TunerSelectOption=Transfer Function Based (PID Tuner App)  InitialConditionSource=internal  InitialConditionForIntegrator=0  InitialConditionForFilter=0  DifferentiatorICPrevScaledInput=0  ExternalReset=none  TrackingMode=off  Kt=1  LimitOutput=off  SatLimitsSource=internal  UpperSaturationLimit=inf  LowerSaturationLimit=-inf  LinearizeAsGain=off  AntiWindupMode=none  Kb=1  POutMin=[]  POutMax=[]  IOutMin=[]  IOutMax=[]  DOutMin=[]  DOutMax=[]  NOutMin=[]  NOutMax=[]  bOutMin=[]  bOutMax=[]  cOutMin=[]  cOutMax=[]  SumOutMin=[]  SumOutMax=[]  SaturationOutMin=[]  SaturationOutMax=[]  PParamMin=[]  PParamMax=[]  IParamMin=[]  IParamMax=[]  DParamMin=[]  DParamMax=[]  NParamMin=[]  NParamMax=[]  bParamMin=[]  bParamMax=[]  cParamMin=[]  cParamMax=[]  KbParamMin=[]  KbParamMax=[]  KtParamMin=[]  KtParamMax=[]  KbOutMin=[]  KbOutMax=[]  KtOutMin=[]  KtOutMax=[]  IntegratorOutMin=[]  IntegratorOutMax=[]  FilterOutMin=[]  FilterOutMax=[]  SumI1OutMin=[]  SumI1OutMax=[]  SumI2OutMin=[]  SumI2OutMax=[]  SumI3OutMin=[]  SumI3OutMax=[]  SumI4OutMin=[]  SumI4OutMax=[]  SumDOutMin=[]  SumDOutMax=[]  Sum1OutMin=[]  Sum1OutMax=[]  Sum2OutMin=[]  Sum2OutMax=[]  Sum3OutMin=[]  Sum3OutMax=[]  DifferentiatorOutMin=[]  DifferentiatorOutMax=[]  FilterDiffOutCoefMin=[]  FilterDiffOutCoefMax=[]  ReciprocalOutMin=[]  ReciprocalOutMax=[]  SumDenOutMin=[]  SumDenOutMax=[]  SumNumOutMin=[]  SumNumOutMax=[]  DivideOutMin=[]  DivideOutMax=[]  UdiffTsProdOutMin=[]  UdiffTsProdOutMax=[]  NTsProdOutMin=[]  NTsProdOutMax=[]  UintegralTsProdOutMin=[]  UintegralTsProdOutMax=[]  UngainTsProdOutMin=[]  UngainTsProdOutMax=[]  IntegratorContinuousStateAttributes=''  IntegratorStateMustResolveToSignalObject=off  IntegratorRTWStateStorageClass=Auto  FilterContinuousStateAttributes=''  FilterStateMustResolveToSignalObject=off  FilterRTWStateStorageClass=Auto  ParallelPVariant=InternalParameters  IdealPVariant=Disabled  IVariant=InternalParameters  DVariant=InternalParameters  bVariant=InternalParameters  cVariant=InternalParameters  IntegratorVariant=Discrete  SatVariant=Disabled  AWVariant=Passthrough  PCopyVariant=Disabled  TRVariant=Disabled  FdbkBlocksVariant=Forward  IdealPFdbkVariant=Disabled  SatFdbkVariant=Disabled  DerivativeFilterVariant=ForwardEulerFilter  NVariant=InternalParameters  NCopyVariant=Disabled  FilterICVariant=InternalICsFilter  IntegratorICVariant=InternalICs  ExternalResetVariant=Disabled  TRSumVariant=Passthrough  SumFdbkVariant=Disabled  SumVariant=Sum_PID  TsampFilterVariant=InternalTs  TsampNgainVariant=Passthrough  TsampIntegralVariant=Passthrough  ExternalSaturationOutDataTypeStr=Inherit: Same as second input
      settings: SourceProductBaseCode=SL
  cfblk5 : Reshape
  cfblk6 : Reshape
  cfblk7 : Constant  Value=[577877722.170944]  SampleTime=1
  cfblk8 : Constant  Value=[-72470325.912385]  SampleTime=1
  cfblk9 : Subsystem
  cfblk2 : Outport
  wires:
  cfblk9/1(cfblk2) -> cfblk6/1
  cfblk3/1 -> cfblk5/1
  cfblk5/1 -> cfblk9/1(cfblk1)
  cfblk4/1 -> cfblk3/1
  cfblk1/1 -> cfblk2/1, cfblk4/2
  cfblk6/1 -> cfblk10/1(cfblk1)
  cfblk8/1 -> cfblk9/2(cfblk6)
  cfblk11/1 -> cfblk9/3(cfblk7)
  cfblk7/1 -> cfblk10/2(cfblk10)
  cfblk10/1(cfblk2) -> cfblk12/1, cfblk13/1
  cfblk12/1 -> cfblk9/4(cfblk8)
  cfblk13/1 -> cfblk4/1

== system sampleModel106/cfblk76/cfblk5 ==
  cfblk1 : Inport
  cfblk7 : Inport  Port=2
  cfblk3 : DiscreteFir  SampleTime=1
  cfblk4 : simulink/Discrete/Transfer Fcn Lead or Lag  PoleZ=0.95  ZeroZ=0.75  ICPrevOutput=0.0  ICPrevInput=0.0  DoSatur=off
      settings: SourceProductBaseCode=SL
  cfblk5 : ComplexToMagnitudeAngle
  cfblk6 : Subsystem
  cfblk8 : Delay  SampleTime=1
  cfblk9 : Delay  SampleTime=1
  cfblk2 : Outport
  wires:
  cfblk6/1(cfblk2) -> cfblk5/1
  cfblk4/1 -> cfblk6/1(cfblk1)
  cfblk7/1 -> cfblk2/1
  cfblk1/1 -> cfblk3/1
  cfblk5/1 -> cfblk8/1
  cfblk8/1 -> cfblk6/2(cfblk10)
  cfblk6/2(cfblk11) -> cfblk9/1
  cfblk9/1 -> cfblk4/1

== system sampleModel106/cfblk76/cfblk6 ==
  cfblk1 : Inport
  cfblk3 : simulink/Discrete/Difference  ICPrevInput=0.0  OutMin=[]  OutMax=[]  OutDataTypeStr=Inherit: Inherit via back propagation  OutDataType=fixdt(1, 16)  OutScaling=2^-10  DoSatur=off
  cfblk4 : DiscreteZeroPole  Poles=[0 0.5]  Gain=1
  cfblk5 : Abs  SaturateOnIntegerOverflow=off
  cfblk6 : UnaryMinus
  cfblk7 : Squeeze
  cfblk8 : Constant  Value=[648448290.023648]  SampleTime=1
  cfblk2 : Outport
  wires:
  cfblk6/1 -> cfblk4/1
  cfblk1/1 -> cfblk5/1
  cfblk3/1 -> cfblk2/1
  cfblk7/1 -> cfblk3/1
  cfblk8/1 -> cfblk6/1
  cfblk5/1 -> cfblk7/1

== system sampleModel106/cfblk76/cfblk7 ==
  cfblk1 : Inport
  cfblk9 : Inport  Port=2
  cfblk10 : Inport  Port=3
  cfblk11 : Inport  Port=4
  cfblk12 : Inport  Port=5
  cfblk3 : slpidlib/PID Controller (2DOF)  Controller=PID  Form=Parallel  TimeDomain=Discrete-time  UseExternalTs=off  SampleTime=1  IntegratorMethod=Forward Euler  FilterMethod=Forward Euler  ControllerParametersSource=internal  P=1  I=1  UseKiTs=off  D=0  N=100  UseFilter=on  b=1  c=1  TunerSelectOption=Transfer Function Based (PID Tuner App)  InitialConditionSource=internal  InitialConditionForIntegrator=0  InitialConditionForFilter=0  DifferentiatorICPrevScaledInput=0  ExternalReset=none  TrackingMode=off  Kt=1  LimitOutput=off  SatLimitsSource=internal  UpperSaturationLimit=inf  LowerSaturationLimit=-inf  LinearizeAsGain=off  AntiWindupMode=none  Kb=1  POutMin=[]  POutMax=[]  IOutMin=[]  IOutMax=[]  DOutMin=[]  DOutMax=[]  NOutMin=[]  NOutMax=[]  bOutMin=[]  bOutMax=[]  cOutMin=[]  cOutMax=[]  SumOutMin=[]  SumOutMax=[]  SaturationOutMin=[]  SaturationOutMax=[]  PParamMin=[]  PParamMax=[]  IParamMin=[]  IParamMax=[]  DParamMin=[]  DParamMax=[]  NParamMin=[]  NParamMax=[]  bParamMin=[]  bParamMax=[]  cParamMin=[]  cParamMax=[]  KbParamMin=[]  KbParamMax=[]  KtParamMin=[]  KtParamMax=[]  KbOutMin=[]  KbOutMax=[]  KtOutMin=[]  KtOutMax=[]  IntegratorOutMin=[]  IntegratorOutMax=[]  FilterOutMin=[]  FilterOutMax=[]  SumI1OutMin=[]  SumI1OutMax=[]  SumI2OutMin=[]  SumI2OutMax=[]  SumI3OutMin=[]  SumI3OutMax=[]  SumI4OutMin=[]  SumI4OutMax=[]  SumDOutMin=[]  SumDOutMax=[]  Sum1OutMin=[]  Sum1OutMax=[]  Sum2OutMin=[]  Sum2OutMax=[]  Sum3OutMin=[]  Sum3OutMax=[]  DifferentiatorOutMin=[]  DifferentiatorOutMax=[]  FilterDiffOutCoefMin=[]  FilterDiffOutCoefMax=[]  ReciprocalOutMin=[]  ReciprocalOutMax=[]  SumDenOutMin=[]  SumDenOutMax=[]  SumNumOutMin=[]  SumNumOutMax=[]  DivideOutMin=[]  DivideOutMax=[]  UdiffTsProdOutMin=[]  UdiffTsProdOutMax=[]  NTsProdOutMin=[]  NTsProdOutMax=[]  UintegralTsProdOutMin=[]  UintegralTsProdOutMax=[]  UngainTsProdOutMin=[]  UngainTsProdOutMax=[]  IntegratorContinuousStateAttributes=''  IntegratorStateMustResolveToSignalObject=off  IntegratorRTWStateStorageClass=Auto  FilterContinuousStateAttributes=''  FilterStateMustResolveToSignalObject=off  FilterRTWStateStorageClass=Auto  ParallelPVariant=InternalParameters  IdealPVariant=Disabled  IVariant=InternalParameters  DVariant=InternalParameters  bVariant=InternalParameters  cVariant=InternalParameters  IntegratorVariant=Discrete  SatVariant=Disabled  AWVariant=Passthrough  PCopyVariant=Disabled  TRVariant=Disabled  FdbkBlocksVariant=Forward  IdealPFdbkVariant=Disabled  SatFdbkVariant=Disabled  DerivativeFilterVariant=ForwardEulerFilter  NVariant=InternalParameters  NCopyVariant=Disabled  FilterICVariant=InternalICsFilter  IntegratorICVariant=InternalICs  ExternalResetVariant=Disabled  TRSumVariant=Passthrough  SumFdbkVariant=Disabled  SumVariant=Sum_PID  TsampFilterVariant=InternalTs  TsampNgainVariant=Passthrough  TsampIntegralVariant=Passthrough  ExternalSaturationOutDataTypeStr=Inherit: Same as second input
      settings: SourceProductBaseCode=SL
  cfblk4 : Squeeze
  cfblk5 : Abs  SaturateOnIntegerOverflow=off
  cfblk6 : Constant  Value=[877841111.447095]  SampleTime=1
  cfblk7 : Constant  Value=[542350248.707149]  SampleTime=1
  cfblk8 : Subsystem
  cfblk2 : Outport
  wires:
  cfblk3/1 -> cfblk8/1(cfblk1)
  cfblk5/1 -> cfblk3/1
  cfblk10/1 -> cfblk2/1
  cfblk6/1 -> cfblk5/1
  cfblk11/1 -> cfblk3/2
  cfblk1/1 -> cfblk4/1

== system sampleModel106/cfblk77/cfblk11 ==
  cfblk1 : Inport
  cfblk7 : Inport  Port=2
  cfblk8 : Inport  Port=3
  cfblk9 : Inport  Port=4
  cfblk10 : Inport  Port=5
  Action Port : ActionPort  ActionPortLabel=if(u1 >= 0)
  cfblk3 : ComplexToMagnitudeAngle
  cfblk4 : Constant  Value=[-625491086.151094]  SampleTime=1
  cfblk5 : Subsystem
  cfblk6 : Subsystem
  cfblk2 : Outport
  wires:
  cfblk7/1 -> cfblk6/1(cfblk1)
  cfblk10/1 -> cfblk2/1
  cfblk4/1 -> cfblk5/1(cfblk1)
  cfblk5/1(cfblk2) -> cfblk6/2(cfblk14)
  cfblk9/1 -> cfblk3/1

== system sampleModel106/cfblk77/cfblk12 ==
  cfblk1 : Inport
  Action Port : ActionPort  ActionPortLabel=else
  cfblk3 : Squeeze
  cfblk4 : Product  Inputs=*
  cfblk5 : Constant  Value=[-232819467.681642]  SampleTime=1
  cfblk6 : Subsystem
  cfblk2 : Outport
  cfblk7 : Outport  Port=2
  wires:
  cfblk5/1 -> cfblk3/1
  cfblk3/1 -> cfblk4/1
  cfblk6/1(cfblk2) -> cfblk2/1
  cfblk4/1 -> cfblk7/1
  cfblk1/1 -> cfblk6/1(cfblk1)

== system sampleModel106/cfblk78/cfblk11 ==
  cfblk1 : Inport
  cfblk8 : Inport  Port=2
  cfblk9 : Inport  Port=3
  Action Port : ActionPort  ActionPortLabel=if(u1 >= 0)
  cfblk11 : Delay
  cfblk3 : DiscreteZeroPole  Poles=[0 0.5]  Gain=1  SampleTime=-1
  cfblk4 : UnitDelay  SampleTime=-1  HasFrameUpgradeWarning=on
  cfblk5 : Constant  Value=[-387919751.020320]  SampleTime=1
  cfblk6 : Subsystem
  cfblk7 : Subsystem
  cfblk2 : Outport
  cfblk10 : Outport  Port=2
  wires:
  cfblk3/1 -> cfblk6/1(cfblk1)
  cfblk9/1 -> cfblk3/1
  cfblk5/1 -> cfblk4/1
  cfblk8/1 -> cfblk2/1
  cfblk4/1 -> cfblk10/1
  cfblk1/1 -> cfblk7/2(cfblk13)
  cfblk7/1(cfblk2) -> cfblk6/2(cfblk16)
  cfblk7/2(cfblk14) -> cfblk6/3(cfblk17)
  cfblk6/1(cfblk2) -> cfblk11/1
  cfblk11/1 -> cfblk7/1(cfblk1)
